simulink model "Boeing787_Yue"  (R2013a)
settings: Solver=ode23tb  SolverMode=SingleTasking  StartTime=0.0  StopTime=346  RelTol=1e-3
InitFcn:
  | load('SampleOutput.mat')
  | 
  | load('SampleFuelBurn.mat')
values from neighbouring files (symbols this model uses):
  FuelBurn = [0 0 0 0 0 0 0 0 0 0 0 0 ... (18249 elements, 1x18249)]    [Benchmark_data1.mat]
undefined symbols (not defined in the file or in its folder): ailerons, AirProp, B_737, elevator, HydProp, landing_gear, rudder, thrust_rev
libraries: PowerFlowLib x118, simulink x20
(part 22 of 26)

== system Boeing787_Yue/Hydraulic/Right Hydraulic System/DC Speed Servo ==
  T_load (Nm) : Inport
  Speed_ref (RPM) : Inport  Port=2
  Voltage : Inport  Port=3
  DC Machine : Subsystem
  Fcn : Fcn  Expr=u(1)/(u(2)+0.1)
  Gain2 : Gain  Gain=60/(2*pi)
  Mux : Mux  Inputs=2
  PID Controller : simulink/Continuous/PID Controller  Controller=PID  TimeDomain=Continuous-time  SampleTime=1  IntegratorMethod=Forward Euler  FilterMethod=Forward Euler  Form=Parallel  P=1  I=0.1  D=0  N=100  InitialConditionSource=internal  InitialConditionForIntegrator=0  InitialConditionForFilter=0  ExternalReset=none  LimitOutput=off  UpperSaturationLimit=inf  LowerSaturationLimit=-inf  LinearizeAsGain=on  AntiWindupMode=none  Kb=1  TrackingMode=off  Kt=1  PParamMin=[]  PParamMax=[]  IParamMin=[]  IParamMax=[]  DParamMin=[]  DParamMax=[]  NParamMin=[]  NParamMax=[]  KbParamMin=[]  KbParamMax=[]  KtParamMin=[]  KtParamMax=[]  POutMin=[]  POutMax=[]  IOutMin=[]  IOutMax=[]  DOutMin=[]  DOutMax=[]  NOutMin=[]  NOutMax=[]  KbOutMin=[]  KbOutMax=[]  KtOutMin=[]  KtOutMax=[]  IntegratorOutMin=[]  IntegratorOutMax=[]  FilterOutMin=[]  FilterOutMax=[]  SumOutMin=[]  SumOutMax=[]  SumI1OutMin=[]  SumI1OutMax=[]  SumI2OutMin=[]  SumI2OutMax=[]  SumI3OutMin=[]  SumI3OutMax=[]  SumDOutMin=[]  SumDOutMax=[]  SaturationOutMin=[]  SaturationOutMax=[]  IntegratorContinuousStateAttributes=''  IntegratorStateMustResolveToSignalObject=off  IntegratorRTWStateStorageClass=Auto  FilterContinuousStateAttributes=''  FilterStateMustResolveToSignalObject=off  FilterRTWStateStorageClass=Auto
  Sum : Sum  Inputs=-+|
  Terminator{,1..3} (4 alike) : Terminator
  w_m : Outport
  i_load : Outport  Port=2
  T_em : Outport  Port=3
  Ploss : Outport  Port=4
  wires:
  DC Machine/5(Plosses) -> Ploss/1
  Sum/1 -> PID Controller/1
  Gain2/1 -> Sum/1, w_m/1
  Speed_ref (RPM)/1 -> Sum/2
  T_load (Nm)/1 -> DC Machine/3(Tload)
  DC Machine/6(Te) -> T_em/1
  Mux/1 -> Fcn/1
  DC Machine/3(Pe) -> Mux/1
  Fcn/1 -> i_load/1
  DC Machine/7(Speed) -> Gain2/1
  Voltage/1 -> DC Machine/1(Vf), Mux/2
  PID Controller/1 -> DC Machine/2(Va)
  DC Machine/8(theta) -> Terminator3/1
  DC Machine/1(If) -> Terminator/1
  DC Machine/2(Ia) -> Terminator1/1
  DC Machine/4(Pm) -> Terminator2/1

== system Boeing787_Yue/Hydraulic/Right Hydraulic System/Sinks ==
  "Motor PLoss " : Inport
  Motor Current Load : Inport  Port=2
  Out1 : Outport
  wires:
  "Motor PLoss "/1 -> Out1/1

== system Boeing787_Yue/ECS/Left Pack/DC Speed Servo1/DC Machine ==
  note: Armature Current ia
  note: Field Current If
  Vf : Inport
  Va : Inport  Port=2
  Tload : Inport  Port=3
  Gain : Gain  Gain=Rfsh
  Gain1 : Gain  Gain=1/Lfsh
  Gain2 : Gain  Gain=Ra
  Gain3 : Gain  Gain=1/La
  Gain4 : Gain  Gain=1/J
  Gain7 : Gain  Gain=Lmsh
  Gain8 : Gain  Gain=Ra
  Gain9 : Gain  Gain=Rfsh
  Integrator : Integrator
  Integrator1 : Integrator
  Integrator2 : Integrator  InitialCondition=1  LimitOutput=on  LowerSaturationLimit=1
  Integrator3 : Integrator  ZeroCross=off
  Math Function1 : Math  Operator=square  SaturateOnIntegerOverflow=on
  Math Function2 : Math  Operator=square  SaturateOnIntegerOverflow=on
  Product{,1..4} (5 alike) : Product  RndMeth=Zero
  Scope : Scope
      settings: SaveName=ScopeData3
  Sum : Sum  Inputs=|+-
  Sum1 : Sum  Inputs=-+-
  Sum2 : Sum  Inputs=+-
  Sum4 : Sum  Inputs=|++
  Sum5 : Sum  Inputs=|++
  Terminator : Terminator
  If : Outport
  Ia : Outport  Port=2
  Pe : Outport  Port=3
  Pm : Outport  Port=4
  Plosses : Outport  Port=5
  Te : Outport  Port=6
  Speed : Outport  Port=7
  theta : Outport  Port=8
  wires:
  Integrator3/1 -> Terminator/1, theta/1
  Gain/1 -> Sum/2
  Sum/1 -> Gain1/1
  Integrator/1 -> Gain/1, [field_ct], If/1
  Sum1/1 -> Gain3/1
  Gain3/1 -> Integrator1/1
  Integrator1/1 -> Gain2/1, [arm_ct], Ia/1
  Product1/1 -> Scope/1, Sum2/1, Te/1
  Sum2/1 -> Gain4/1
  Gain4/1 -> Integrator2/1
  Gain1/1 -> Integrator/1
  Product/1 -> Sum1/1
  Gain2/1 -> Sum1/3
  [lambdaf] -> Product1/1
  [arm_ct] -> Product1/2
  [load_torque] -> Sum2/2
  [speed] -> Product/2
  [lambdaf] -> Product/1
  [field_ct] -> Gain7/1
  Gain7/1 -> [lambdaf]
  Vf/1 -> Sum/1, [vf]
  Va/1 -> Sum1/2, [va]
  [va] -> Product2/1
  [arm_ct] -> Product2/2
  Product2/1 -> Sum4/1
  [vf] -> Product3/1
  [field_ct] -> Product3/2
  Product3/1 -> Sum4/2
  Sum4/1 -> Pe/1
  [load_torque] -> Product4/1
  [speed] -> Product4/2
  Product4/1 -> Pm/1
  [arm_ct] -> Math Function1/1
  Math Function1/1 -> Gain8/1
  Gain8/1 -> Sum5/1
  [field_ct] -> Math Function2/1
  Math Function2/1 -> Gain9/1
  Gain9/1 -> Sum5/2
  Sum5/1 -> Plosses/1
  Integrator2/1 -> Speed/1, [speed], Integrator3/1
  Tload/1 -> [load_torque]

== system Boeing787_Yue/ECS/Left Pack/DC Speed Servo2/DC Machine ==
  note: Armature Current ia
  note: Field Current If
  Vf : Inport
  Va : Inport  Port=2
  Tload : Inport  Port=3
  Gain : Gain  Gain=Rfsh
  Gain1 : Gain  Gain=1/Lfsh
  Gain2 : Gain  Gain=Ra
  Gain3 : Gain  Gain=1/La
  Gain4 : Gain  Gain=1/J
  Gain7 : Gain  Gain=Lmsh
  Gain8 : Gain  Gain=Ra
  Gain9 : Gain  Gain=Rfsh
  Integrator : Integrator
  Integrator1 : Integrator
  Integrator2 : Integrator  InitialCondition=1  LimitOutput=on  LowerSaturationLimit=1
  Integrator3 : Integrator  ZeroCross=off
  Math Function1 : Math  Operator=square  SaturateOnIntegerOverflow=on
  Math Function2 : Math  Operator=square  SaturateOnIntegerOverflow=on
  Product{,1..4} (5 alike) : Product  RndMeth=Zero
  Scope : Scope
      settings: SaveName=ScopeData3
  Sum : Sum  Inputs=|+-
  Sum1 : Sum  Inputs=-+-
  Sum2 : Sum  Inputs=+-
  Sum4 : Sum  Inputs=|++
  Sum5 : Sum  Inputs=|++
  Terminator : Terminator
  If : Outport
  Ia : Outport  Port=2
  Pe : Outport  Port=3
  Pm : Outport  Port=4
  Plosses : Outport  Port=5
  Te : Outport  Port=6
  Speed : Outport  Port=7
  theta : Outport  Port=8
  wires:
  Integrator3/1 -> Terminator/1, theta/1
  Gain/1 -> Sum/2
  Sum/1 -> Gain1/1
  Integrator/1 -> Gain/1, [field_ct], If/1
  Sum1/1 -> Gain3/1
  Gain3/1 -> Integrator1/1
  Integrator1/1 -> Gain2/1, [arm_ct], Ia/1
  Product1/1 -> Scope/1, Sum2/1, Te/1
  Sum2/1 -> Gain4/1
  Gain4/1 -> Integrator2/1
  Gain1/1 -> Integrator/1
  Product/1 -> Sum1/1
  Gain2/1 -> Sum1/3
  [lambdaf] -> Product1/1
  [arm_ct] -> Product1/2
  [load_torque] -> Sum2/2
  [speed] -> Product/2
  [lambdaf] -> Product/1
  [field_ct] -> Gain7/1
  Gain7/1 -> [lambdaf]
  Vf/1 -> Sum/1, [vf]
  Va/1 -> Sum1/2, [va]
  [va] -> Product2/1
  [arm_ct] -> Product2/2
  Product2/1 -> Sum4/1
  [vf] -> Product3/1
  [field_ct] -> Product3/2
  Product3/1 -> Sum4/2
  Sum4/1 -> Pe/1
  [load_torque] -> Product4/1
  [speed] -> Product4/2
  Product4/1 -> Pm/1
  [arm_ct] -> Math Function1/1
  Math Function1/1 -> Gain8/1
  Gain8/1 -> Sum5/1
  [field_ct] -> Math Function2/1
  Math Function2/1 -> Gain9/1
  Gain9/1 -> Sum5/2
  Sum5/1 -> Plosses/1
  Integrator2/1 -> Speed/1, [speed], Integrator3/1
  Tload/1 -> [load_torque]

== system Boeing787_Yue/ECS/Left Pack/Primary HX (air-air)/Air_properties_in_flows_hot_and_cold ==
  In_flow_bus_hot : Inport
  In_flow_bus_cold : Inport  Port=2
  Bus Creator : BusCreator  Inputs=5
  Bus Creator3 : BusCreator  Inputs=5
  air_properties_in_cold : Subsystem
  air_properties_in_hot : Subsystem
  air_properties_in_hot1 : Outport
  air_properties_in_cold1 : Outport  Port=2
  wires:
  air_properties_in_hot/4(K_air_Wm-1K-2) -> Bus Creator/4  "K_air"
  air_properties_in_cold/5(Pr) -> Bus Creator3/5  "Pr"
  air_properties_in_hot/5(Pr) -> Bus Creator/5  "Pr"
  In_flow_bus_cold/1 -> air_properties_in_cold/1(In_flow_bus_cold)
  In_flow_bus_hot/1 -> air_properties_in_hot/1(In_flow_bus_hot)
  Bus Creator/1 -> air_properties_in_hot1/1
  Bus Creator3/1 -> air_properties_in_cold1/1
  air_properties_in_hot/3(mu_air_Pa.s) -> Bus Creator/3  "mu_air"
  air_properties_in_hot/2(cp_air_Jkg-1K-1) -> Bus Creator/2  "cp_air"
  air_properties_in_hot/1(rho_air_kgm-3) -> Bus Creator/1  "rho_air"
  air_properties_in_cold/4(K_air_Wm-1K-2) -> Bus Creator3/4  "K_air"
  air_properties_in_cold/3(mu_air_Pa.s) -> Bus Creator3/3  "mu_air"
  air_properties_in_cold/2(cp_air_Jkg-1K-1) -> Bus Creator3/2  "cp_air"
  air_properties_in_cold/1(rho_air_kgm-3) -> Bus Creator3/1  "rho_air"

== system Boeing787_Yue/ECS/Left Pack/Primary HX (air-air)/C_T_c_av ==
  In_flow_bus : Inport
  air_properties : Inport  Port=2
  Tot_thermal_resist : Inport  Port=3
  Add : Sum
  Bus Selector : BusSelector  OutputSignals=mdot_kgps
  Bus Selector1 : BusSelector  OutputSignals=cp_air
  Constant : Constant
  Divide : Product  Inputs=***
  Divide1 : Product  Inputs=*/
  Gain : Gain  Gain=2
  C_T_c_av : Outport
  wires:
  Divide1/1 -> C_T_c_av/1
  Add/1 -> Divide1/2
  Constant/1 -> Add/2
  Gain/1 -> Divide1/1, Add/1
  Divide/1 -> Gain/1
  Bus Selector1/1 -> Divide/3  "<cp_air>"
  Bus Selector/1 -> Divide/2  "<mdot_kgps>"
  Tot_thermal_resist/1 -> Divide/1  "R_tot_c"
  In_flow_bus/1 -> Bus Selector/1
  air_properties/1 -> Bus Selector1/1

== system Boeing787_Yue/ECS/Left Pack/Primary HX (air-air)/C_T_c_i ==
  In_flow_bus : Inport
  air_properties : Inport  Port=2
  Tot_thermal_resist : Inport  Port=3
  HX_parameters : Inport  Port=4
  Add : Sum
  Bus Selector : BusSelector  OutputSignals=mdot_kgps
  Bus Selector1 : BusSelector  OutputSignals=cp_air
  Bus Selector2 : BusSelector  OutputSignals=m_cm,cp_hx
  Constant : Constant
  Divide : Product  Inputs=***
  Divide2 : Product  Inputs=**///
  Gain : Gain  Gain=2
  Gain1 : Gain  Gain=2
  C_T_c_i : Outport
  wires:
  In_flow_bus/1 -> Bus Selector/1
  air_properties/1 -> Bus Selector1/1
  Tot_thermal_resist/1 -> Divide/1  "R_tot"
  Bus Selector/1 -> Divide/2, Divide2/1  "<mdot_kgps>"
  Bus Selector1/1 -> Divide/3, Divide2/2  "<cp_air>"
  Divide/1 -> Gain/1
  Gain/1 -> Add/1
  Constant/1 -> Add/2
  HX_parameters/1 -> Bus Selector2/1
  Bus Selector2/1 -> Divide2/3  "<m_cm>"
  Bus Selector2/2 -> Divide2/4  "<cp_hx>"
  Add/1 -> Divide2/5
  Gain1/1 -> C_T_c_i/1
  Divide2/1 -> Gain1/1

== system Boeing787_Yue/ECS/Left Pack/Primary HX (air-air)/C_T_h_av ==
  In_flow_bus : Inport
  air_properties : Inport  Port=2
  Tot_thermal_resist : Inport  Port=3
  Add : Sum
  Bus Selector : BusSelector  OutputSignals=mdot_kgps
  Bus Selector1 : BusSelector  OutputSignals=cp_air
  Constant : Constant
  Divide : Product  Inputs=***
  Divide1 : Product  Inputs=*/
  Gain : Gain  Gain=2
  C_T_h_av : Outport
  wires:
  Divide1/1 -> C_T_h_av/1
  Add/1 -> Divide1/2
  Constant/1 -> Add/2
  Gain/1 -> Divide1/1, Add/1
  Divide/1 -> Gain/1
  Bus Selector1/1 -> Divide/3  "<cp_air>"
  Bus Selector/1 -> Divide/2  "<mdot_kgps>"
  Tot_thermal_resist/1 -> Divide/1  "R_tot_h"
  In_flow_bus/1 -> Bus Selector/1
  air_properties/1 -> Bus Selector1/1

== system Boeing787_Yue/ECS/Left Pack/Primary HX (air-air)/C_T_h_i ==
  In_flow_bus : Inport
  air_properties : Inport  Port=2
  Tot_thermal_resist : Inport  Port=3
  HX_parameters : Inport  Port=4
  Add : Sum
  Bus Selector : BusSelector  OutputSignals=mdot_kgps
  Bus Selector1 : BusSelector  OutputSignals=cp_air
  Bus Selector2 : BusSelector  OutputSignals=m_cm,cp_hx
  Constant : Constant
  Divide : Product  Inputs=***
  Divide2 : Product  Inputs=**///
  Gain : Gain  Gain=2
  Gain1 : Gain  Gain=2
  C_T_h_i : Outport
  wires:
  Gain1/1 -> C_T_h_i/1
  Add/1 -> Divide2/5
  Bus Selector2/2 -> Divide2/4  "<cp_hx>"
  Bus Selector2/1 -> Divide2/3  "<m_cm>"
  HX_parameters/1 -> Bus Selector2/1
  Constant/1 -> Add/2
  Gain/1 -> Add/1
  Divide/1 -> Gain/1
  Bus Selector1/1 -> Divide/3, Divide2/2  "<cp_air>"
  Bus Selector/1 -> Divide/2, Divide2/1  "<mdot_kgps>"
  Tot_thermal_resist/1 -> Divide/1  "R_tot_h"
  air_properties/1 -> Bus Selector1/1
  In_flow_bus/1 -> Bus Selector/1
  Divide2/1 -> Gain1/1

== system Boeing787_Yue/ECS/Left Pack/Primary HX (air-air)/Calculating_T_c_av ==
  T_cm : Inport
  In_flow_bus : Inport  Port=2
  C_t_c_av : Inport  Port=3
  Add1 : Sum  Inputs=-+
  Add3 : Sum
  Bus Selector : BusSelector  OutputSignals=temp_C
  Divide1 : Product  Inputs=**
  T_c_av_degreC : Outport
  wires:
  T_cm/1 -> Add3/1, Add1/1  "T_cm"
  In_flow_bus/1 -> Bus Selector/1
  Bus Selector/1 -> Add1/2  "<temp_C>"
  C_t_c_av/1 -> Divide1/2
  Add1/1 -> Divide1/1  "T_c_i - T_cm"
  Divide1/1 -> Add3/2
  Add3/1 -> T_c_av_degreC/1

== system Boeing787_Yue/ECS/Left Pack/Primary HX (air-air)/Calculating_T_h_av ==
  T_cm : Inport
  In_flow_bus : Inport  Port=2
  C_t_h_av : Inport  Port=3
  Add1 : Sum  Inputs=-+
  Add3 : Sum
  Bus Selector : BusSelector  OutputSignals=temp_C
  Divide1 : Product  Inputs=**
  T_h_av_degreC : Outport
  wires:
  Add1/1 -> Divide1/1  "T_h_i - T_cm"
  C_t_h_av/1 -> Divide1/2
  Bus Selector/1 -> Add1/2  "<temp_C>"
  In_flow_bus/1 -> Bus Selector/1
  T_cm/1 -> Add1/1, Add3/1  "T_cm"
  Add3/1 -> T_h_av_degreC/1
  Divide1/1 -> Add3/2

== system Boeing787_Yue/ECS/Left Pack/Primary HX (air-air)/Calculating_core_mass_temp ==
  note: dTcm/dt
  note: Tcm
  C_T_h_i : Inport
  C_T_c_i : Inport  Port=2
  C_t_cm : Inport  Port=3
  In_flow_bus_hot : Inport  Port=4
  In_flow_bus_cold : Inport  Port=5
  Add : Sum  Inputs=++-
  Bus Selector : BusSelector  OutputSignals=temp_C
  Bus Selector1 : BusSelector  OutputSignals=temp_C
  Divide : Product  Inputs=**
  Divide1 : Product  Inputs=**
  Divide2 : Product  Inputs=**
  Integrator : Integrator  InitialCondition=T_cm_0
  Core_mass_temp_C : Outport
  wires:
  Divide1/1 -> Add/3
  C_t_cm/1 -> Divide1/2
  Integrator/1 -> Core_mass_temp_C/1, Divide1/1
  Add/1 -> Integrator/1
  Divide2/1 -> Add/2
  Divide/1 -> Add/1
  Bus Selector1/1 -> Divide2/2  "<temp_C>"
  C_T_c_i/1 -> Divide2/1
  Bus Selector/1 -> Divide/2  "<temp_C>"
  C_T_h_i/1 -> Divide/1
  In_flow_bus_cold/1 -> Bus Selector1/1
  In_flow_bus_hot/1 -> Bus Selector/1

== system Boeing787_Yue/ECS/Left Pack/Primary HX (air-air)/Colburn_J_factor_cold ==
  Fin_prameter_ratios : Inport
  Re : Inport  Port=2
  Add : Sum
  Bus Selector : BusSelector  OutputSignals=alpha_fin,delta_fin,gamma_fin
  Constant : Constant  Value=-0.5403
  Constant1 : Constant  Value=-0.1541
  Constant2 : Constant  Value=0.1499
  Constant3 : Constant  Value=-0.0678
  Constant4 : Constant  Value=1.34
  Constant5 : Constant  Value=0.504
  Constant6 : Constant  Value=0.456
  Constant7 : Constant  Value=-1.055
  Constant8 : Constant
  Constant9 : Constant  Value=0.1
  Divide : Product  Inputs=****
  Divide1 : Product  Inputs=****
  Divide2 : Product  Inputs=**
  Gain : Gain  Gain=0.6522
  Gain1 : Gain  Gain=5.269*10^(-5)
  Re1 : Math  Operator=pow  SaturateOnIntegerOverflow=on
  Re2 : Math  Operator=pow  SaturateOnIntegerOverflow=on
  alpha_fin : Math  Operator=pow  SaturateOnIntegerOverflow=on
  alpha_fin1 : Math  Operator=pow  SaturateOnIntegerOverflow=on
  delta_fin : Math  Operator=pow  SaturateOnIntegerOverflow=on
  delta_fin1 : Math  Operator=pow  SaturateOnIntegerOverflow=on
  gamma_fin : Math  Operator=pow  SaturateOnIntegerOverflow=on
  gamma_fin1 : Math  Operator=pow  SaturateOnIntegerOverflow=on
  gamma_fin2 : Math  Operator=pow  SaturateOnIntegerOverflow=on
  Colburn_J_factor : Outport
  wires:
  Divide2/1 -> Colburn_J_factor/1
  Gain/1 -> Divide2/1
  gamma_fin2/1 -> Divide2/2
  Constant9/1 -> gamma_fin2/2
  Add/1 -> gamma_fin2/1
  Gain1/1 -> Add/1
  Constant8/1 -> Add/2
  Divide1/1 -> Gain1/1
  gamma_fin1/1 -> Divide1/4
  delta_fin1/1 -> Divide1/3
  alpha_fin1/1 -> Divide1/2
  Re2/1 -> Divide1/1
  Divide/1 -> Gain/1
  gamma_fin/1 -> Divide/4
  delta_fin/1 -> Divide/3
  alpha_fin/1 -> Divide/2
  Re1/1 -> Divide/1
  Bus Selector/3 -> gamma_fin1/1, gamma_fin/1  "<gamma_fin>"
  Bus Selector/2 -> delta_fin1/1, delta_fin/1  "<delta_fin>"
  Bus Selector/1 -> alpha_fin1/1, alpha_fin/1  "<alpha_fin>"
  Re/1 -> Re2/1, Re1/1
  Constant7/1 -> gamma_fin1/2
  Constant6/1 -> delta_fin1/2
  Constant5/1 -> alpha_fin1/2
  Constant4/1 -> Re2/2
  Constant3/1 -> gamma_fin/2
  Constant2/1 -> delta_fin/2
  Constant1/1 -> alpha_fin/2
  Constant/1 -> Re1/2
  Fin_prameter_ratios/1 -> Bus Selector/1

== system Boeing787_Yue/ECS/Left Pack/Primary HX (air-air)/Colburn_J_factor_hot ==
  Fin_prameter_ratios : Inport
  Re : Inport  Port=2
  Add : Sum
  Bus Selector : BusSelector  OutputSignals=alpha_fin,delta_fin,gamma_fin
  Constant : Constant  Value=-0.5403
  Constant1 : Constant  Value=-0.1541
  Constant2 : Constant  Value=0.1499
  Constant3 : Constant  Value=-0.0678
  Constant4 : Constant  Value=1.34
  Constant5 : Constant  Value=0.504
  Constant6 : Constant  Value=0.456
  Constant7 : Constant  Value=-1.055
  Constant8 : Constant
  Constant9 : Constant  Value=0.1
  Divide : Product  Inputs=****
  Divide1 : Product  Inputs=****
  Divide2 : Product  Inputs=**
  Gain : Gain  Gain=0.6522
  Gain1 : Gain  Gain=5.269*10^(-5)
  Re1 : Math  Operator=pow  SaturateOnIntegerOverflow=on
  Re2 : Math  Operator=pow  SaturateOnIntegerOverflow=on
  alpha_fin : Math  Operator=pow  SaturateOnIntegerOverflow=on
  alpha_fin1 : Math  Operator=pow  SaturateOnIntegerOverflow=on
  delta_fin : Math  Operator=pow  SaturateOnIntegerOverflow=on
  delta_fin1 : Math  Operator=pow  SaturateOnIntegerOverflow=on
  gamma_fin : Math  Operator=pow  SaturateOnIntegerOverflow=on
  gamma_fin1 : Math  Operator=pow  SaturateOnIntegerOverflow=on
  gamma_fin2 : Math  Operator=pow  SaturateOnIntegerOverflow=on
  Colburn_J_factor : Outport
  wires:
  Fin_prameter_ratios/1 -> Bus Selector/1
  Constant/1 -> Re1/2
  Constant1/1 -> alpha_fin/2
  Constant2/1 -> delta_fin/2
  Constant3/1 -> gamma_fin/2
  Constant4/1 -> Re2/2
  Constant5/1 -> alpha_fin1/2
  Constant6/1 -> delta_fin1/2
  Constant7/1 -> gamma_fin1/2
  Re/1 -> Re1/1, Re2/1
  Bus Selector/1 -> alpha_fin/1, alpha_fin1/1  "<alpha_fin>"
  Bus Selector/2 -> delta_fin/1, delta_fin1/1  "<delta_fin>"
  Bus Selector/3 -> gamma_fin/1, gamma_fin1/1  "<gamma_fin>"
  Re1/1 -> Divide/1
  alpha_fin/1 -> Divide/2
  delta_fin/1 -> Divide/3
  gamma_fin/1 -> Divide/4
  Divide/1 -> Gain/1
  Re2/1 -> Divide1/1
  alpha_fin1/1 -> Divide1/2
  delta_fin1/1 -> Divide1/3
  gamma_fin1/1 -> Divide1/4
  Divide1/1 -> Gain1/1
  Constant8/1 -> Add/2
  Gain1/1 -> Add/1
  Add/1 -> gamma_fin2/1
  Constant9/1 -> gamma_fin2/2
  gamma_fin2/1 -> Divide2/2
  Gain/1 -> Divide2/1
  Divide2/1 -> Colburn_J_factor/1

== system Boeing787_Yue/ECS/Left Pack/Primary HX (air-air)/Friction_factor_cold ==
  Fin_prameter_ratios : Inport
  Re : Inport  Port=2
  Add : Sum
  Bus Selector : BusSelector  OutputSignals=alpha_fin,delta_fin,gamma_fin
  Constant : Constant  Value=-0.7422
  Constant1 : Constant  Value=-0.1856
  Constant2 : Constant  Value=0.3053
  Constant3 : Constant  Value=-0.2659
  Constant4 : Constant  Value=4.429
  Constant5 : Constant  Value=0.92
  Constant6 : Constant  Value=3.767
  Constant7 : Constant  Value=0.236
  Constant8 : Constant
  Constant9 : Constant  Value=0.1
  Divide : Product  Inputs=****
  Divide1 : Product  Inputs=****
  Divide2 : Product  Inputs=**
  Gain : Gain  Gain=9.6243
  Gain1 : Gain  Gain=7.669*10^(-8)
  Re1 : Math  Operator=pow  SaturateOnIntegerOverflow=on
  Re2 : Math  Operator=pow  SaturateOnIntegerOverflow=on
  alpha_fin : Math  Operator=pow  SaturateOnIntegerOverflow=on
  alpha_fin1 : Math  Operator=pow  SaturateOnIntegerOverflow=on
  delta_fin : Math  Operator=pow  SaturateOnIntegerOverflow=on
  delta_fin1 : Math  Operator=pow  SaturateOnIntegerOverflow=on
  gamma_fin : Math  Operator=pow  SaturateOnIntegerOverflow=on
  gamma_fin1 : Math  Operator=pow  SaturateOnIntegerOverflow=on
  gamma_fin2 : Math  Operator=pow  SaturateOnIntegerOverflow=on
  Friction_factor : Outport
  wires:
  Fin_prameter_ratios/1 -> Bus Selector/1
  Constant/1 -> Re1/2
  Constant1/1 -> alpha_fin/2
  Constant2/1 -> delta_fin/2
  Constant3/1 -> gamma_fin/2
  Constant4/1 -> Re2/2
  Constant5/1 -> alpha_fin1/2
  Constant6/1 -> delta_fin1/2
  Constant7/1 -> gamma_fin1/2
  Re/1 -> Re1/1, Re2/1
  Bus Selector/1 -> alpha_fin/1, alpha_fin1/1  "<alpha_fin>"
  Bus Selector/2 -> delta_fin/1, delta_fin1/1  "<delta_fin>"
  Bus Selector/3 -> gamma_fin/1, gamma_fin1/1  "<gamma_fin>"
  Re1/1 -> Divide/1
  alpha_fin/1 -> Divide/2
  delta_fin/1 -> Divide/3
  gamma_fin/1 -> Divide/4
  Divide/1 -> Gain/1
  Re2/1 -> Divide1/1
  alpha_fin1/1 -> Divide1/2
  delta_fin1/1 -> Divide1/3
  gamma_fin1/1 -> Divide1/4
  Divide1/1 -> Gain1/1
  Constant8/1 -> Add/2
  Gain1/1 -> Add/1
  Add/1 -> gamma_fin2/1
  Constant9/1 -> gamma_fin2/2
  gamma_fin2/1 -> Divide2/2
  Gain/1 -> Divide2/1
  Divide2/1 -> Friction_factor/1

== system Boeing787_Yue/ECS/Left Pack/Primary HX (air-air)/Friction_factor_hot ==
  Fin_prameter_ratios : Inport
  Re : Inport  Port=2
  Add : Sum
  Bus Selector : BusSelector  OutputSignals=alpha_fin,delta_fin,gamma_fin
  Constant : Constant  Value=-0.7422
  Constant1 : Constant  Value=-0.1856
  Constant2 : Constant  Value=0.3053
  Constant3 : Constant  Value=-0.2659
  Constant4 : Constant  Value=4.429
  Constant5 : Constant  Value=0.92
  Constant6 : Constant  Value=3.767
  Constant7 : Constant  Value=0.236
  Constant8 : Constant
  Constant9 : Constant  Value=0.1
  Divide : Product  Inputs=****
  Divide1 : Product  Inputs=****
  Divide2 : Product  Inputs=**
  Gain : Gain  Gain=9.6243
  Gain1 : Gain  Gain=7.669*10^(-8)
  Re1 : Math  Operator=pow  SaturateOnIntegerOverflow=on
  Re2 : Math  Operator=pow  SaturateOnIntegerOverflow=on
  alpha_fin : Math  Operator=pow  SaturateOnIntegerOverflow=on
  alpha_fin1 : Math  Operator=pow  SaturateOnIntegerOverflow=on
  delta_fin : Math  Operator=pow  SaturateOnIntegerOverflow=on
  delta_fin1 : Math  Operator=pow  SaturateOnIntegerOverflow=on
  gamma_fin : Math  Operator=pow  SaturateOnIntegerOverflow=on
  gamma_fin1 : Math  Operator=pow  SaturateOnIntegerOverflow=on
  gamma_fin2 : Math  Operator=pow  SaturateOnIntegerOverflow=on
  Friction_factor : Outport
  wires:
  Divide2/1 -> Friction_factor/1
  Gain/1 -> Divide2/1
  gamma_fin2/1 -> Divide2/2
  Constant9/1 -> gamma_fin2/2
  Add/1 -> gamma_fin2/1
  Gain1/1 -> Add/1
  Constant8/1 -> Add/2
  Divide1/1 -> Gain1/1
  gamma_fin1/1 -> Divide1/4
  delta_fin1/1 -> Divide1/3
  alpha_fin1/1 -> Divide1/2
  Re2/1 -> Divide1/1
  Divide/1 -> Gain/1
  gamma_fin/1 -> Divide/4
  delta_fin/1 -> Divide/3
  alpha_fin/1 -> Divide/2
  Re1/1 -> Divide/1
  Bus Selector/3 -> gamma_fin1/1, gamma_fin/1  "<gamma_fin>"
  Bus Selector/2 -> delta_fin1/1, delta_fin/1  "<delta_fin>"
  Bus Selector/1 -> alpha_fin1/1, alpha_fin/1  "<alpha_fin>"
  Re/1 -> Re2/1, Re1/1
  Constant7/1 -> gamma_fin1/2
  Constant6/1 -> delta_fin1/2
  Constant5/1 -> alpha_fin1/2
  Constant4/1 -> Re2/2
  Constant3/1 -> gamma_fin/2
  Constant2/1 -> delta_fin/2
  Constant1/1 -> alpha_fin/2
  Constant/1 -> Re1/2
  Fin_prameter_ratios/1 -> Bus Selector/1

== system Boeing787_Yue/ECS/Left Pack/Primary HX (air-air)/HX_and_Fin_paramters ==
  Bus Creator1 : BusCreator  Inputs=6
  Bus Creator2 : BusCreator  Inputs=6
  Bus Creator3 : BusCreator  Inputs=3
  Fin_parameters : Subsystem
  HX_parameters : Subsystem
  Other_HX_parameters2 : Subsystem
  alpha : Product  Inputs=*/
  delta : Product  Inputs=*/
  gamma : Product  Inputs=*/
  HX_parameters2 : Outport
  Fin_parameters1 : Outport  Port=2
  Fin_parameters_ratios : Outport  Port=3
  wires:
  [Other_HX_parameters] -> HX_parameters/1(Other_HX_parameters)
  Other_HX_parameters2/1(Out1) -> [Other_HX_parameters]
  Bus Creator3/1 -> Fin_parameters_ratios/1
  gamma/1 -> Bus Creator3/3  "gamma_fin"
  delta/1 -> Bus Creator3/2  "delta_fin"
  alpha/1 -> Bus Creator3/1  "alpha_fin"
  Bus Creator1/1 -> HX_parameters2/1
  Bus Creator2/1 -> HX_parameters/2(Fin_parameters), Fin_parameters1/1
  HX_parameters/1(tot_free_flow_area_m^2) -> Bus Creator1/1  "A"
  Fin_parameters/3(Fin_free_flow_width_m) -> Bus Creator2/3, alpha/1, gamma/2  "s_fin"
  Fin_parameters/6(Fin_eff) -> Bus Creator2/6  "eta_fin"
  Fin_parameters/5(K_fin_Wm-1K-1) -> Bus Creator2/5  "K_n"
  Fin_parameters/4(Fin_free_flow_height_m) -> Bus Creator2/4, alpha/2  "h_fin"
  Fin_parameters/2(Fin_thickness_m) -> gamma/1, Bus Creator2/2, delta/1  "t_fin"
  Fin_parameters/1(Fin_length_m) -> Bus Creator2/1, delta/2  "l_fin"
  HX_parameters/6(m_hx_kg) -> Bus Creator1/6  "m_cm"
  HX_parameters/5(cp_hx_Jkg-1K-1) -> Bus Creator1/5  "cp_hx"
  HX_parameters/4(K_hx_Wm-1K-1) -> Bus Creator1/4  "K_p"
  HX_parameters/3(tot_no_of_fins_per_HX_per_flow) -> Bus Creator1/3  "N_f"
  HX_parameters/2(tot_length_in_direc_of_flow_m) -> Bus Creator1/2  "L_hx"

== system Boeing787_Yue/ECS/Left Pack/Primary HX (air-air)/Heat_load_cold_side ==
  In_flow_bus : Inport
  air_properties : Inport  Port=2
  temp_out_degreeC : Inport  Port=3
  Bus Selector : BusSelector  OutputSignals=temp_C,mdot_kgps
  Bus Selector1 : BusSelector  OutputSignals=cp_air
  Product : Product  Inputs=3  RndMeth=Zero
  temp_diff : Sum  Inputs=-+
  Heat_rate_Watt : Outport
  wires:
  In_flow_bus/1 -> Bus Selector/1
  air_properties/1 -> Bus Selector1/1
  Bus Selector/1 -> temp_diff/1  "<temp_C>"
  temp_out_degreeC/1 -> temp_diff/2
  Bus Selector/2 -> Product/1  "<mdot_kgps>"
  Bus Selector1/1 -> Product/2  "<cp_air>"
  temp_diff/1 -> Product/3
  Product/1 -> Heat_rate_Watt/1

== system Boeing787_Yue/ECS/Left Pack/Primary HX (air-air)/Heat_load_hot_side ==
  In_flow_bus : Inport
  air_properties : Inport  Port=2
  temp_out_degreeC : Inport  Port=3
  Bus Selector : BusSelector  OutputSignals=temp_C,mdot_kgps
  Bus Selector1 : BusSelector  OutputSignals=cp_air
  Product : Product  Inputs=3  RndMeth=Zero
  temp_diff : Sum  Inputs=+-
  Heat_rate_Watt : Outport
  wires:
  Product/1 -> Heat_rate_Watt/1
  temp_diff/1 -> Product/3
  Bus Selector1/1 -> Product/2  "<cp_air>"
  Bus Selector/2 -> Product/1  "<mdot_kgps>"
  temp_out_degreeC/1 -> temp_diff/2
  Bus Selector/1 -> temp_diff/1  "<temp_C>"
  air_properties/1 -> Bus Selector1/1
  In_flow_bus/1 -> Bus Selector/1

== system Boeing787_Yue/ECS/Left Pack/Primary HX (air-air)/Hydraulic_diam_m ==
  Fin_parameters : Inport
  Add : Sum  Inputs=+++
  Add1 : Sum
  Bus Selector1 : BusSelector  OutputSignals=l_fin,t_fin,s_fin,h_fin,K_n,eta_fin
  Gain : Gain  Gain=4
  Gain1 : Gain  Gain=2
  Terminator : Terminator
  Terminator1 : Terminator
  hl : Product  Inputs=**
  shl : Product  Inputs=***
  sl : Product  Inputs=**
  th : Product  Inputs=**
  ts : Product  Inputs=**
  ts1 : Product  Inputs=*/
  Out1 : Outport
  wires:
  ts1/1 -> Out1/1
  Add1/1 -> ts1/2
  Gain/1 -> ts1/1
  ts/1 -> Add1/2
  Gain1/1 -> Add1/1
  Add/1 -> Gain1/1
  th/1 -> Add/3
  hl/1 -> Add/2
  sl/1 -> Add/1
  Bus Selector1/2 -> th/1, ts/1  "<t_fin>"
  shl/1 -> Gain/1
  Bus Selector1/1 -> hl/2, sl/2, shl/3  "<l_fin>"
  Bus Selector1/4 -> th/2, shl/2, hl/1  "<h_fin>"
  Bus Selector1/3 -> ts/2, sl/1, shl/1  "<s_fin>"
  Fin_parameters/1 -> Bus Selector1/1
  Bus Selector1/5 -> Terminator/1  "<K_n>"
  Bus Selector1/6 -> Terminator1/1  "<eta_fin>"

== system Boeing787_Yue/ECS/Left Pack/Primary HX (air-air)/Pressure_drop_cold ==
  Friction_factor : Inport
  HX_parameters : Inport  Port=2
  air_properties : Inport  Port=3
  air_velocity : Inport  Port=4
  D_hydraulic : Inport  Port=5
  In_flow_bus : Inport  Port=6
  Add : Sum  Inputs=-+
  Bus Selector : BusSelector  OutputSignals=L_hx
  Bus Selector1 : BusSelector  OutputSignals=rho_air
  Bus Selector2 : BusSelector  OutputSignals=press_Pa
  Constant : Constant  Value=2
  Divide3 : Product  Inputs=****/
  Gain2 : Gain  Gain=2
  Math Function : Math  Operator=pow  SaturateOnIntegerOverflow=on
  pres_drop_Pa : Outport
  pres_Pa : Outport  Port=2
  wires:
  Friction_factor/1 -> Divide3/1
  HX_parameters/1 -> Bus Selector/1
  Bus Selector/1 -> Divide3/2  "<L_hx>"
  air_properties/1 -> Bus Selector1/1
  Bus Selector1/1 -> Divide3/3  "<rho_air>"
  air_velocity/1 -> Math Function/1
  Constant/1 -> Math Function/2
  Math Function/1 -> Divide3/4
  D_hydraulic/1 -> Divide3/5
  Divide3/1 -> Gain2/1
  Gain2/1 -> pres_drop_Pa/1, Add/1  "pres_drop_Pa"
  In_flow_bus/1 -> Bus Selector2/1
  Bus Selector2/1 -> Add/2  "<press_Pa>"
  Add/1 -> pres_Pa/1

== system Boeing787_Yue/ECS/Left Pack/Primary HX (air-air)/Pressure_drop_hot ==
  Friction_factor : Inport
  HX_parameters : Inport  Port=2
  air_properties : Inport  Port=3
  air_velocity : Inport  Port=4
  D_hydraulic : Inport  Port=5
  In_flow_bus : Inport  Port=6
  Add : Sum  Inputs=-+
  Bus Selector : BusSelector  OutputSignals=L_hx
  Bus Selector1 : BusSelector  OutputSignals=rho_air
  Bus Selector2 : BusSelector  OutputSignals=pres_Pa
  Constant : Constant  Value=2
  Divide3 : Product  Inputs=****/
  Gain2 : Gain  Gain=2
  Math Function : Math  Operator=pow  SaturateOnIntegerOverflow=on
  pres_drop_Pa : Outport
  pres_Pa : Outport  Port=2
  wires:
  Add/1 -> pres_Pa/1
  Bus Selector2/1 -> Add/2  "<pres_Pa>"
  In_flow_bus/1 -> Bus Selector2/1
  Gain2/1 -> Add/1, pres_drop_Pa/1  "pres_drop_Pa"
  Divide3/1 -> Gain2/1
  D_hydraulic/1 -> Divide3/5
  Math Function/1 -> Divide3/4
  Constant/1 -> Math Function/2
  air_velocity/1 -> Math Function/1
  Bus Selector1/1 -> Divide3/3  "<rho_air>"
  air_properties/1 -> Bus Selector1/1
  Bus Selector/1 -> Divide3/2  "<L_hx>"
  HX_parameters/1 -> Bus Selector/1
  Friction_factor/1 -> Divide3/1

== system Boeing787_Yue/ECS/Left Pack/Primary HX (air-air)/Re_number_in_cold ==
  In_flow_bus : Inport
  air_properties : Inport  Port=2
  Hydraulic_diam : Inport  Port=3
  HX_paramters : Inport  Port=4
  Bus Selector : BusSelector  OutputSignals=mdot_kgps
  Bus Selector1 : BusSelector  OutputSignals=rho_air,mu_air
  Bus Selector2 : BusSelector  OutputSignals=A
  Re_number_claculation : Product  Inputs=***/
  Velocity_calculation : Product  Inputs=*//
  Re_number : Outport
  velo_air_ms-1 : Outport  Port=2
  wires:
  air_properties/1 -> Bus Selector1/1
  In_flow_bus/1 -> Bus Selector/1
  HX_paramters/1 -> Bus Selector2/1
  Bus Selector/1 -> Velocity_calculation/1  "<mdot_kgps>"
  Bus Selector1/1 -> Velocity_calculation/2, Re_number_claculation/1  "<rho_air>"
  Bus Selector2/1 -> Velocity_calculation/3  "<A>"
  Velocity_calculation/1 -> velo_air_ms-1/1, Re_number_claculation/2  "Velo_air_ms-1"
  Hydraulic_diam/1 -> Re_number_claculation/3
  Bus Selector1/2 -> Re_number_claculation/4  "<mu_air>"
  Re_number_claculation/1 -> Re_number/1  "Re_number"

== system Boeing787_Yue/ECS/Left Pack/Primary HX (air-air)/Re_number_in_hot ==
  In_flow_bus : Inport
  air_properties : Inport  Port=2
  Hydraulic_diam : Inport  Port=3
  HX_paramters : Inport  Port=4
  Bus Selector : BusSelector  OutputSignals=mdot_kgps
  Bus Selector1 : BusSelector  OutputSignals=rho_air,mu_air
  Bus Selector2 : BusSelector  OutputSignals=A
  Re_number_claculation : Product  Inputs=***/
  Velocity_calculation : Product  Inputs=*//
  Re_number : Outport
  velo_air_ms-1 : Outport  Port=2
  wires:
  Re_number_claculation/1 -> Re_number/1  "Re_number"
  Bus Selector1/2 -> Re_number_claculation/4  "<mu_air>"
  Hydraulic_diam/1 -> Re_number_claculation/3
  Velocity_calculation/1 -> velo_air_ms-1/1, Re_number_claculation/2  "Velo_air_ms-1"
  Bus Selector2/1 -> Velocity_calculation/3  "<A>"
  Bus Selector1/1 -> Re_number_claculation/1, Velocity_calculation/2  "<rho_air>"
  Bus Selector/1 -> Velocity_calculation/1  "<mdot_kgps>"
  HX_paramters/1 -> Bus Selector2/1
  In_flow_bus/1 -> Bus Selector/1
  air_properties/1 -> Bus Selector1/1

== system Boeing787_Yue/ECS/Left Pack/Primary HX (air-air)/Thermal_resistance_KpW_cold ==
  Convective_HTC : Inport
  HX_parameters : Inport  Port=2
  Fin_parameters : Inport  Port=3
  Add : Sum
  Bus Selector : BusSelector  OutputSignals=N_f
  Bus Selector1 : BusSelector  OutputSignals=s_fin,l_fin,eta_fin,h_fin
  Calc_R_tot : Product  Inputs=**
  Calc_R_tot1 : Product  Inputs=*/
  Constant : Constant  Value=2
  Gain : Gain  Gain=2
  R1_Convection_to_plate/fin_base : Product  Inputs=////
  R1_convection_fin_or_plate_base_KpW : Display
  R5_Conv-conduction_through fin_projection : Product  Inputs=//////
  R5_convection_fin_projection_KpW : Display
  R_tot_K/W : Outport
  wires:
  HX_parameters/1 -> Bus Selector/1
  Fin_parameters/1 -> Bus Selector1/1
  Convective_HTC/1 -> R1_Convection_to_plate/fin_base/1, R5_Conv-conduction_through fin_projection/3  "HTC_Wpm2K"
  Bus Selector/1 -> R1_Convection_to_plate/fin_base/2, R5_Conv-conduction_through fin_projection/4  "<N_f>"
  Bus Selector1/1 -> R1_Convection_to_plate/fin_base/3  "<s_fin>"
  Bus Selector1/2 -> R1_Convection_to_plate/fin_base/4, R5_Conv-conduction_through fin_projection/6  "<l_fin>"
  R1_Convection_to_plate/fin_base/1 -> R1_convection_fin_or_plate_base_KpW/1, Calc_R_tot/1, Add/1
  Constant/1 -> R5_Conv-conduction_through fin_projection/1
  Bus Selector1/3 -> R5_Conv-conduction_through fin_projection/2  "<eta_fin>"
  Bus Selector1/4 -> R5_Conv-conduction_through fin_projection/5  "<h_fin>"
  R5_Conv-conduction_through fin_projection/1 -> R5_convection_fin_projection_KpW/1, Calc_R_tot/2, Gain/1
  Gain/1 -> Add/2
  Calc_R_tot/1 -> Calc_R_tot1/1  "R1R5"
  Add/1 -> Calc_R_tot1/2  "R1+2R5"
  Calc_R_tot1/1 -> R_tot_K/W/1  "Rtot"

== system Boeing787_Yue/ECS/Left Pack/Primary HX (air-air)/Thermal_resistance_KpW_hot ==
  Convective_HTC : Inport
  HX_parameters : Inport  Port=2
  Fin_parameters : Inport  Port=3
  Add : Sum
  Bus Selector : BusSelector  OutputSignals=N_f
  Bus Selector1 : BusSelector  OutputSignals=s_fin,l_fin,eta_fin,h_fin
  Calc_R_tot : Product  Inputs=**
  Calc_R_tot1 : Product  Inputs=*/
  Constant : Constant  Value=2
  Gain : Gain  Gain=2
  R1_Convection_to_plate/fin_base : Product  Inputs=////
  R1_convection_fin_or_plate_base_KpW : Display
  R5_Conv-conduction_through fin_projection : Product  Inputs=//////
  R5_convection_fin_projection_KpW : Display
  R_tot_K/W : Outport
  wires:
  Calc_R_tot1/1 -> R_tot_K/W/1  "Rtot"
  Add/1 -> Calc_R_tot1/2  "R1+2R5"
  Calc_R_tot/1 -> Calc_R_tot1/1  "R1R5"
  Gain/1 -> Add/2
  R5_Conv-conduction_through fin_projection/1 -> Gain/1, Calc_R_tot/2, R5_convection_fin_projection_KpW/1
  Bus Selector1/4 -> R5_Conv-conduction_through fin_projection/5  "<h_fin>"
  Bus Selector1/3 -> R5_Conv-conduction_through fin_projection/2  "<eta_fin>"
  Constant/1 -> R5_Conv-conduction_through fin_projection/1
  R1_Convection_to_plate/fin_base/1 -> Add/1, Calc_R_tot/1, R1_convection_fin_or_plate_base_KpW/1
  Bus Selector1/2 -> R5_Conv-conduction_through fin_projection/6, R1_Convection_to_plate/fin_base/4  "<l_fin>"
  Bus Selector1/1 -> R1_Convection_to_plate/fin_base/3  "<s_fin>"
  Bus Selector/1 -> R5_Conv-conduction_through fin_projection/4, R1_Convection_to_plate/fin_base/2  "<N_f>"
  Convective_HTC/1 -> R5_Conv-conduction_through fin_projection/3, R1_Convection_to_plate/fin_base/1  "HTC_Wpm2K"
  Fin_parameters/1 -> Bus Selector1/1
  HX_parameters/1 -> Bus Selector/1

== system Boeing787_Yue/ECS/Left Pack/Primary HX (air-air)/convective_HTC_Wm-2K-1_cold ==
  Colburn_J_factor : Inport
  Re : Inport  Port=2
  air_properties : Inport  Port=3
  hydraulic_diameter : Inport  Port=4
  Bus Selector : BusSelector  OutputSignals=Pr,K_air
  Constant : Constant  Value=1/3
  Divide : Product  Inputs=****/
  Math Function : Math  Operator=pow  SaturateOnIntegerOverflow=on
  Convective_HTC_Wm-2K-1 : Outport
  wires:
  air_properties/1 -> Bus Selector/1
  Colburn_J_factor/1 -> Divide/1
  Re/1 -> Divide/2
  Bus Selector/1 -> Math Function/1  "<Pr>"
  Constant/1 -> Math Function/2
  Math Function/1 -> Divide/3
  Bus Selector/2 -> Divide/4  "<K_air>"
  hydraulic_diameter/1 -> Divide/5
  Divide/1 -> Convective_HTC_Wm-2K-1/1

== system Boeing787_Yue/ECS/Left Pack/Primary HX (air-air)/convective_HTC_Wm-2K-1_hot ==
  Colburn_J_factor : Inport
  Re : Inport  Port=2
  air_properties : Inport  Port=3
  hydraulic_diameter : Inport  Port=4
  Bus Selector : BusSelector  OutputSignals=Pr,K_air
  Constant : Constant  Value=1/3
  Divide : Product  Inputs=****/
  Math Function : Math  Operator=pow  SaturateOnIntegerOverflow=on
  Convective_HTC_Wm-2K-1 : Outport
  wires:
  Divide/1 -> Convective_HTC_Wm-2K-1/1
  hydraulic_diameter/1 -> Divide/5
  Bus Selector/2 -> Divide/4  "<K_air>"
  Math Function/1 -> Divide/3
  Constant/1 -> Math Function/2
  Bus Selector/1 -> Math Function/1  "<Pr>"
  Re/1 -> Divide/2
  Colburn_J_factor/1 -> Divide/1
  air_properties/1 -> Bus Selector/1

== system Boeing787_Yue/ECS/Left Pack/Secondary HX (air-air)1/Air_properties_in_flows_hot_and_cold ==
  In_flow_bus_hot : Inport
  In_flow_bus_cold : Inport  Port=2
  Bus Creator : BusCreator  Inputs=5
  Bus Creator3 : BusCreator  Inputs=5
  air_properties_in_cold : Subsystem
  air_properties_in_hot : Subsystem
  air_properties_in_hot1 : Outport
  air_properties_in_cold1 : Outport  Port=2
  wires:
  air_properties_in_hot/4(K_air_Wm-1K-2) -> Bus Creator/4  "K_air"
  air_properties_in_cold/5(Pr) -> Bus Creator3/5  "Pr"
  air_properties_in_hot/5(Pr) -> Bus Creator/5  "Pr"
  In_flow_bus_cold/1 -> air_properties_in_cold/1(In_flow_bus_cold)
  In_flow_bus_hot/1 -> air_properties_in_hot/1(In_flow_bus_hot)
  Bus Creator/1 -> air_properties_in_hot1/1
  Bus Creator3/1 -> air_properties_in_cold1/1
  air_properties_in_hot/3(mu_air_Pa.s) -> Bus Creator/3  "mu_air"
  air_properties_in_hot/2(cp_air_Jkg-1K-1) -> Bus Creator/2  "cp_air"
  air_properties_in_hot/1(rho_air_kgm-3) -> Bus Creator/1  "rho_air"
  air_properties_in_cold/4(K_air_Wm-1K-2) -> Bus Creator3/4  "K_air"
  air_properties_in_cold/3(mu_air_Pa.s) -> Bus Creator3/3  "mu_air"
  air_properties_in_cold/2(cp_air_Jkg-1K-1) -> Bus Creator3/2  "cp_air"
  air_properties_in_cold/1(rho_air_kgm-3) -> Bus Creator3/1  "rho_air"

== system Boeing787_Yue/ECS/Left Pack/Secondary HX (air-air)1/C_T_c_av ==
  In_flow_bus : Inport
  air_properties : Inport  Port=2
  Tot_thermal_resist : Inport  Port=3
  Add : Sum
  Bus Selector : BusSelector  OutputSignals=mdot_kgps
  Bus Selector1 : BusSelector  OutputSignals=cp_air
  Constant : Constant
  Divide : Product  Inputs=***
  Divide1 : Product  Inputs=*/
  Gain : Gain  Gain=2
  C_T_c_av : Outport
  wires:
  Divide1/1 -> C_T_c_av/1
  Add/1 -> Divide1/2
  Constant/1 -> Add/2
  Gain/1 -> Divide1/1, Add/1
  Divide/1 -> Gain/1
  Bus Selector1/1 -> Divide/3  "<cp_air>"
  Bus Selector/1 -> Divide/2  "<mdot_kgps>"
  Tot_thermal_resist/1 -> Divide/1  "R_tot_c"
  In_flow_bus/1 -> Bus Selector/1
  air_properties/1 -> Bus Selector1/1

== system Boeing787_Yue/ECS/Left Pack/Secondary HX (air-air)1/C_T_c_i ==
  In_flow_bus : Inport
  air_properties : Inport  Port=2
  Tot_thermal_resist : Inport  Port=3
  HX_parameters : Inport  Port=4
  Add : Sum
  Bus Selector : BusSelector  OutputSignals=mdot_kgps
  Bus Selector1 : BusSelector  OutputSignals=cp_air
  Bus Selector2 : BusSelector  OutputSignals=m_cm,cp_hx
  Constant : Constant
  Divide : Product  Inputs=***
  Divide2 : Product  Inputs=**///
  Gain : Gain  Gain=2
  Gain1 : Gain  Gain=2
  C_T_c_i : Outport
  wires:
  In_flow_bus/1 -> Bus Selector/1
  air_properties/1 -> Bus Selector1/1
  Tot_thermal_resist/1 -> Divide/1  "R_tot"
  Bus Selector/1 -> Divide/2, Divide2/1  "<mdot_kgps>"
  Bus Selector1/1 -> Divide/3, Divide2/2  "<cp_air>"
  Divide/1 -> Gain/1
  Gain/1 -> Add/1
  Constant/1 -> Add/2
  HX_parameters/1 -> Bus Selector2/1
  Bus Selector2/1 -> Divide2/3  "<m_cm>"
  Bus Selector2/2 -> Divide2/4  "<cp_hx>"
  Add/1 -> Divide2/5
  Gain1/1 -> C_T_c_i/1
  Divide2/1 -> Gain1/1

== system Boeing787_Yue/ECS/Left Pack/Secondary HX (air-air)1/C_T_h_av ==
  In_flow_bus : Inport
  air_properties : Inport  Port=2
  Tot_thermal_resist : Inport  Port=3
  Add : Sum
  Bus Selector : BusSelector  OutputSignals=mdot_kgps
  Bus Selector1 : BusSelector  OutputSignals=cp_air
  Constant : Constant
  Divide : Product  Inputs=***
  Divide1 : Product  Inputs=*/
  Gain : Gain  Gain=2
  C_T_h_av : Outport
  wires:
  Divide1/1 -> C_T_h_av/1
  Add/1 -> Divide1/2
  Constant/1 -> Add/2
  Gain/1 -> Divide1/1, Add/1
  Divide/1 -> Gain/1
  Bus Selector1/1 -> Divide/3  "<cp_air>"
  Bus Selector/1 -> Divide/2  "<mdot_kgps>"
  Tot_thermal_resist/1 -> Divide/1  "R_tot_h"
  In_flow_bus/1 -> Bus Selector/1
  air_properties/1 -> Bus Selector1/1

== system Boeing787_Yue/ECS/Left Pack/Secondary HX (air-air)1/C_T_h_i ==
  In_flow_bus : Inport
  air_properties : Inport  Port=2
  Tot_thermal_resist : Inport  Port=3
  HX_parameters : Inport  Port=4
  Add : Sum
  Bus Selector : BusSelector  OutputSignals=mdot_kgps
  Bus Selector1 : BusSelector  OutputSignals=cp_air
  Bus Selector2 : BusSelector  OutputSignals=m_cm,cp_hx
  Constant : Constant
  Divide : Product  Inputs=***
  Divide2 : Product  Inputs=**///
  Gain : Gain  Gain=2
  Gain1 : Gain  Gain=2
  C_T_h_i : Outport
  wires:
  Gain1/1 -> C_T_h_i/1
  Add/1 -> Divide2/5
  Bus Selector2/2 -> Divide2/4  "<cp_hx>"
  Bus Selector2/1 -> Divide2/3  "<m_cm>"
  HX_parameters/1 -> Bus Selector2/1
  Constant/1 -> Add/2
  Gain/1 -> Add/1
  Divide/1 -> Gain/1
  Bus Selector1/1 -> Divide/3, Divide2/2  "<cp_air>"
  Bus Selector/1 -> Divide/2, Divide2/1  "<mdot_kgps>"
  Tot_thermal_resist/1 -> Divide/1  "R_tot_h"
  air_properties/1 -> Bus Selector1/1
  In_flow_bus/1 -> Bus Selector/1
  Divide2/1 -> Gain1/1

== system Boeing787_Yue/ECS/Left Pack/Secondary HX (air-air)1/Calculating_T_c_av ==
  T_cm : Inport
  In_flow_bus : Inport  Port=2
  C_t_c_av : Inport  Port=3
  Add1 : Sum  Inputs=-+
  Add3 : Sum
  Bus Selector : BusSelector  OutputSignals=temp_C
  Divide1 : Product  Inputs=**
  T_c_av_degreC : Outport
  wires:
  T_cm/1 -> Add3/1, Add1/1  "T_cm"
  In_flow_bus/1 -> Bus Selector/1
  Bus Selector/1 -> Add1/2  "<temp_C>"
  C_t_c_av/1 -> Divide1/2
  Add1/1 -> Divide1/1  "T_c_i - T_cm"
  Divide1/1 -> Add3/2
  Add3/1 -> T_c_av_degreC/1

== system Boeing787_Yue/ECS/Left Pack/Secondary HX (air-air)1/Calculating_T_h_av ==
  T_cm : Inport
  In_flow_bus : Inport  Port=2
  C_t_h_av : Inport  Port=3
  Add1 : Sum  Inputs=-+
  Add3 : Sum
  Bus Selector : BusSelector  OutputSignals=temp_C
  Divide1 : Product  Inputs=**
  T_h_av_degreC : Outport
  wires:
  Add1/1 -> Divide1/1  "T_h_i - T_cm"
  C_t_h_av/1 -> Divide1/2
  Bus Selector/1 -> Add1/2  "<temp_C>"
  In_flow_bus/1 -> Bus Selector/1
  T_cm/1 -> Add1/1, Add3/1  "T_cm"
  Add3/1 -> T_h_av_degreC/1
  Divide1/1 -> Add3/2

== system Boeing787_Yue/ECS/Left Pack/Secondary HX (air-air)1/Calculating_core_mass_temp ==
  note: dTcm/dt
  note: Tcm
  C_T_h_i : Inport
  C_T_c_i : Inport  Port=2
  C_t_cm : Inport  Port=3
  In_flow_bus_hot : Inport  Port=4
  In_flow_bus_cold : Inport  Port=5
  Add : Sum  Inputs=++-
  Bus Selector : BusSelector  OutputSignals=temp_C
  Bus Selector1 : BusSelector  OutputSignals=temp_C
  Divide : Product  Inputs=**
  Divide1 : Product  Inputs=**
  Divide2 : Product  Inputs=**
  Integrator : Integrator  InitialCondition=T_cm_0
  Core_mass_temp_C : Outport
  wires:
  Divide1/1 -> Add/3
  C_t_cm/1 -> Divide1/2
  Integrator/1 -> Core_mass_temp_C/1, Divide1/1
  Add/1 -> Integrator/1
  Divide2/1 -> Add/2
  Divide/1 -> Add/1
  Bus Selector1/1 -> Divide2/2  "<temp_C>"
  C_T_c_i/1 -> Divide2/1
  Bus Selector/1 -> Divide/2  "<temp_C>"
  C_T_h_i/1 -> Divide/1
  In_flow_bus_cold/1 -> Bus Selector1/1
  In_flow_bus_hot/1 -> Bus Selector/1

== system Boeing787_Yue/ECS/Left Pack/Secondary HX (air-air)1/Colburn_J_factor_cold ==
  Fin_prameter_ratios : Inport
  Re : Inport  Port=2
  Add : Sum
  Bus Selector : BusSelector  OutputSignals=alpha_fin,delta_fin,gamma_fin
  Constant : Constant  Value=-0.5403
  Constant1 : Constant  Value=-0.1541
  Constant2 : Constant  Value=0.1499
  Constant3 : Constant  Value=-0.0678
  Constant4 : Constant  Value=1.34
  Constant5 : Constant  Value=0.504
  Constant6 : Constant  Value=0.456
  Constant7 : Constant  Value=-1.055
  Constant8 : Constant
  Constant9 : Constant  Value=0.1
  Divide : Product  Inputs=****
  Divide1 : Product  Inputs=****
  Divide2 : Product  Inputs=**
  Gain : Gain  Gain=0.6522
  Gain1 : Gain  Gain=5.269*10^(-5)
  Re1 : Math  Operator=pow  SaturateOnIntegerOverflow=on
  Re2 : Math  Operator=pow  SaturateOnIntegerOverflow=on
  alpha_fin : Math  Operator=pow  SaturateOnIntegerOverflow=on
  alpha_fin1 : Math  Operator=pow  SaturateOnIntegerOverflow=on
  delta_fin : Math  Operator=pow  SaturateOnIntegerOverflow=on
  delta_fin1 : Math  Operator=pow  SaturateOnIntegerOverflow=on
  gamma_fin : Math  Operator=pow  SaturateOnIntegerOverflow=on
  gamma_fin1 : Math  Operator=pow  SaturateOnIntegerOverflow=on
  gamma_fin2 : Math  Operator=pow  SaturateOnIntegerOverflow=on
  Colburn_J_factor : Outport
  wires:
  Divide2/1 -> Colburn_J_factor/1
  Gain/1 -> Divide2/1
  gamma_fin2/1 -> Divide2/2
  Constant9/1 -> gamma_fin2/2
  Add/1 -> gamma_fin2/1
  Gain1/1 -> Add/1
  Constant8/1 -> Add/2
  Divide1/1 -> Gain1/1
  gamma_fin1/1 -> Divide1/4
  delta_fin1/1 -> Divide1/3
  alpha_fin1/1 -> Divide1/2
  Re2/1 -> Divide1/1
  Divide/1 -> Gain/1
  gamma_fin/1 -> Divide/4
  delta_fin/1 -> Divide/3
  alpha_fin/1 -> Divide/2
  Re1/1 -> Divide/1
  Bus Selector/3 -> gamma_fin1/1, gamma_fin/1  "<gamma_fin>"
  Bus Selector/2 -> delta_fin1/1, delta_fin/1  "<delta_fin>"
  Bus Selector/1 -> alpha_fin1/1, alpha_fin/1  "<alpha_fin>"
  Re/1 -> Re2/1, Re1/1
  Constant7/1 -> gamma_fin1/2
  Constant6/1 -> delta_fin1/2
  Constant5/1 -> alpha_fin1/2
  Constant4/1 -> Re2/2
  Constant3/1 -> gamma_fin/2
  Constant2/1 -> delta_fin/2
  Constant1/1 -> alpha_fin/2
  Constant/1 -> Re1/2
  Fin_prameter_ratios/1 -> Bus Selector/1

== system Boeing787_Yue/ECS/Left Pack/Secondary HX (air-air)1/Colburn_J_factor_hot ==
  Fin_prameter_ratios : Inport
  Re : Inport  Port=2
  Add : Sum
  Bus Selector : BusSelector  OutputSignals=alpha_fin,delta_fin,gamma_fin
  Constant : Constant  Value=-0.5403
  Constant1 : Constant  Value=-0.1541
  Constant2 : Constant  Value=0.1499
  Constant3 : Constant  Value=-0.0678
  Constant4 : Constant  Value=1.34
  Constant5 : Constant  Value=0.504
  Constant6 : Constant  Value=0.456
  Constant7 : Constant  Value=-1.055
  Constant8 : Constant
  Constant9 : Constant  Value=0.1
  Divide : Product  Inputs=****
  Divide1 : Product  Inputs=****
  Divide2 : Product  Inputs=**
  Gain : Gain  Gain=0.6522
  Gain1 : Gain  Gain=5.269*10^(-5)
  Re1 : Math  Operator=pow  SaturateOnIntegerOverflow=on
  Re2 : Math  Operator=pow  SaturateOnIntegerOverflow=on
  alpha_fin : Math  Operator=pow  SaturateOnIntegerOverflow=on
  alpha_fin1 : Math  Operator=pow  SaturateOnIntegerOverflow=on
  delta_fin : Math  Operator=pow  SaturateOnIntegerOverflow=on
  delta_fin1 : Math  Operator=pow  SaturateOnIntegerOverflow=on
  gamma_fin : Math  Operator=pow  SaturateOnIntegerOverflow=on
  gamma_fin1 : Math  Operator=pow  SaturateOnIntegerOverflow=on
  gamma_fin2 : Math  Operator=pow  SaturateOnIntegerOverflow=on
  Colburn_J_factor : Outport
  wires:
  Fin_prameter_ratios/1 -> Bus Selector/1
  Constant/1 -> Re1/2
  Constant1/1 -> alpha_fin/2
  Constant2/1 -> delta_fin/2
  Constant3/1 -> gamma_fin/2
  Constant4/1 -> Re2/2
  Constant5/1 -> alpha_fin1/2
  Constant6/1 -> delta_fin1/2
  Constant7/1 -> gamma_fin1/2
  Re/1 -> Re1/1, Re2/1
  Bus Selector/1 -> alpha_fin/1, alpha_fin1/1  "<alpha_fin>"
  Bus Selector/2 -> delta_fin/1, delta_fin1/1  "<delta_fin>"
  Bus Selector/3 -> gamma_fin/1, gamma_fin1/1  "<gamma_fin>"
  Re1/1 -> Divide/1
  alpha_fin/1 -> Divide/2
  delta_fin/1 -> Divide/3
  gamma_fin/1 -> Divide/4
  Divide/1 -> Gain/1
  Re2/1 -> Divide1/1
  alpha_fin1/1 -> Divide1/2
  delta_fin1/1 -> Divide1/3
  gamma_fin1/1 -> Divide1/4
  Divide1/1 -> Gain1/1
  Constant8/1 -> Add/2
  Gain1/1 -> Add/1
  Add/1 -> gamma_fin2/1
  Constant9/1 -> gamma_fin2/2
  gamma_fin2/1 -> Divide2/2
  Gain/1 -> Divide2/1
  Divide2/1 -> Colburn_J_factor/1
